simulink model "MySusp_ParasiticFriction_RTW"  (Simulink 9.1)
settings: Solver=ode1  StartTime=0.0  StopTime=inf  FixedStep=0.001  RelTol=1e-3
PreLoadFcn:
  | vehicle = 'Car'; if ~length(which('cmself')), cmenv; end
  | MySusp_ParasiticFriction_RTW_bus
  | MySusp_ParasiticFriction_RTW_params
InitFcn:
  | vehicle = 'Car'; if ~length(which('cmself')), cmenv; end
  | MySusp_ParasiticFriction_RTW_bus
values from neighbouring files (symbols this model uses):
  Damping = 150    [MySusp_ParasiticFriction_RTW_params.m]
  mu_c = 1.0    (= 1)    [MySusp_ParasiticFriction_RTW_params.m]
  PreloadForce = 30    [MySusp_ParasiticFriction_RTW_params.m]
  Stiffness = 50000    [MySusp_ParasiticFriction_RTW_params.m]    (also in MySusp_Spring_RTW_params.m = 5000; MySusp_Stabi_RTW_params.m = 15000)
  v0 = 0.01    [MySusp_ParasiticFriction_RTW_params.m]
Description:
  | CarMaker Plug-in Model Target
settings Model: SuppressorTable=22 serialization::archive 11 0 6 0 0 0 1 0  Creator=ml  LastModifiedBy=ml
settings DataIOCC: SaveFormat=Dataset
settings OptimizationCC: LifeSpan=auto
settings DebuggingCC: UnderspecifiedInitializationDetection=Simplified  MergeDetectMultiDrivingBlocksExec=error  SFUnexpectedBacktrackingDiag=error  SFNoUnconditionalDefaultTransitionDiag=error  SFExecutionAtInitializationDiag=warning
settings HardwareCC: ProdBitPerPointer=64  ProdBitPerSizeT=64  ProdBitPerPtrDiffT=64  ProdLargestAtomicFloat=Float  ProdIntDivRoundTo=Zero  ProdEndianess=LittleEndian  ProdWordSize=64  ProdHWDeviceType=Intel->x86-64 (Windows64)
settings ModelReferenceCC: PropagateSignalLabelsOutOfModel=on
settings RTWCC: SystemTargetFile=CarMaker.tlc  TemplateMakefile=CarMaker_unix-win64.tmf  Description=CarMaker Plug-in Model Target
settings CodeAppCC: MaxIdLength=127
settings STFCustomTargetCC: TargetLangStandard=C99 (ISO)  CombineOutputUpdateFcns=on  MultiInstanceERTCode=on  CodeInterfacePackaging=Reusable function  GRTInterface=off  GenerateAllocFcn=on  SystemTargetFile=CarMaker.tlc
settings GRTTargetCC: TargetLangStandard=C99 (ISO)  ParMdlRefBuildCompliant=off  CompOptLevelCompliant=off  ConcurrentExecutionCompliant=off  CombineOutputUpdateFcns=on  MatFileLogging=off  MultiInstanceERTCode=on  CodeInterfacePackaging=Reusable function  CPPClassGenCompliant=off  GRTInterface=off  GenerateAllocFcn=on  UseToolchainInfoCompliant=off  RTWCAPISignals=on  RTWCAPIParams=on  RTWCAPIStates=on
settings CustomProperty: DataType=string
settings EnumStrPairs: String=Car
settings ConfigComp: CovMetricSettings=dwe  CovHtmlReporting=off  CovSaveCumulativeToWorkspaceVar=off  CovSaveSingleToWorkspaceVar=off  CovExternalEMLEnable=on

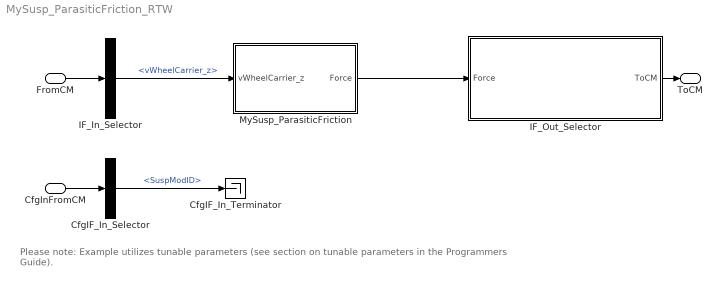
== system MySusp_ParasiticFriction_RTW ==
  note: Please note: Example utilizes tunable parameters (see section on tunable parameters in the Programmers Guide).
  FromCM : Inport  OutDataTypeStr=Bus: cmSusp_ParasiticEffectsIn
  CfgInFromCM : Inport  Port=2  OutDataTypeStr=Bus: cmSusp_ParasiticEffectsCfgIn
  CfgIF_In_Selector : BusSelector  OutputSignals=SuspModID
  CfgIF_In_Terminator : Terminator
  IF_In_Selector : BusSelector  OutputSignals=vWheelCarrier_z
  IF_Out_Selector : Subsystem  mask(Signal Selection){}
      mask help: Signal Selection Block
      settings: OpenFcn=cmSignalSelect('SignalSelection_CB',gcb)
  MySusp_ParasiticFriction : Subsystem
  ToCM : Outport  OutDataTypeStr=Bus: cmSusp_ParasiticEffectsOut
  wires:
  FromCM/1 -> IF_In_Selector/1
  IF_In_Selector/1 -> MySusp_ParasiticFriction/1(vWheelCarrier_z)  "<vWheelCarrier_z>"
  IF_Out_Selector/1(ToCM) -> ToCM/1
  CfgInFromCM/1 -> CfgIF_In_Selector/1
  CfgIF_In_Selector/1 -> CfgIF_In_Terminator/1  "<SuspModID>"
  MySusp_ParasiticFriction/1(Force) -> IF_Out_Selector/1(Force)

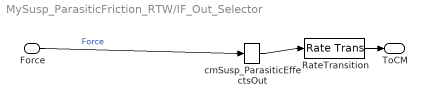
== system MySusp_ParasiticFriction_RTW/IF_Out_Selector ==
  Force : Inport
  RateTransition : RateTransition  OutPortSampleTime=str2num(get_param(bdroot,'FixedStep'))
  cmSusp_ParasiticEffectsOut : BusCreator  Inputs=1
  ToCM : Outport
  wires:
  RateTransition/1 -> ToCM/1
  cmSusp_ParasiticEffectsOut/1 -> RateTransition/1
  Force/1 -> cmSusp_ParasiticEffectsOut/1  "Force"

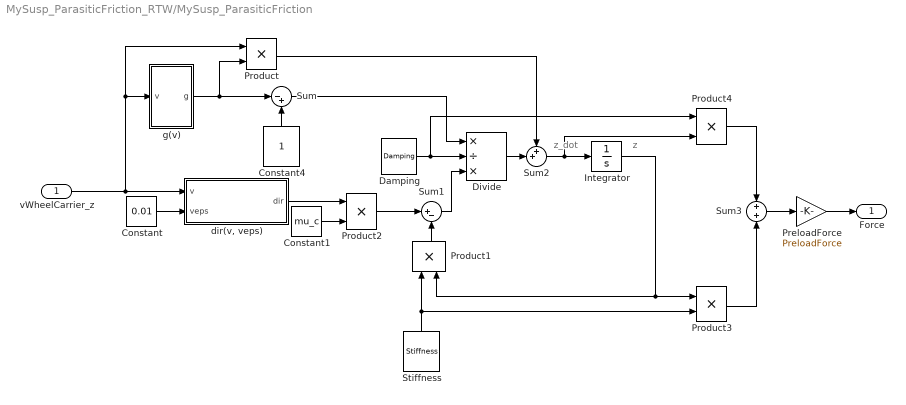
== system MySusp_ParasiticFriction_RTW/MySusp_ParasiticFriction ==
  note: z_dot
  note: z
  vWheelCarrier_z : Inport
  Constant : Constant  Value=0.01
  Constant1 : Constant  Value=mu_c
  Constant4 : Constant
  Damping : Constant  Value=Damping
  Divide : Product  Inputs=*/*
  Integrator : Integrator
  PreloadForce : Gain  Gain=PreloadForce
  Product{,1..4} (5 alike) : Product
  Stiffness : Constant  Value=Stiffness
  Sum : Sum  Inputs=|-+
  Sum1 : Sum  Inputs=|+-
  Sum2 : Sum  Inputs=++|
  Sum3 : Sum
  "dir(v, veps)" : Subsystem
  g(v) : Subsystem
  Force : Outport
  wires:
  Sum3/1 -> PreloadForce/1
  PreloadForce/1 -> Force/1
  Sum/1 -> Divide/1
  Stiffness/1 -> Product1/1, Product3/2
  Sum1/1 -> Divide/3
  Damping/1 -> Product4/1, Divide/2
  Divide/1 -> Sum2/2
  Product/1 -> Sum2/1
  vWheelCarrier_z/1 -> "dir(v, veps)"/1(v), g(v)/1(v), Product/1
  Constant/1 -> "dir(v, veps)"/2(veps)
  g(v)/1(g) -> Sum/1, Product/2
  Constant1/1 -> Product2/2
  "dir(v, veps)"/1(dir) -> Product2/1
  Product2/1 -> Sum1/1
  Constant4/1 -> Sum/2
  Sum2/1 -> Product4/2, Integrator/1
  Integrator/1 -> Product1/2, Product3/1
  Product1/1 -> Sum1/2
  Product3/1 -> Sum3/2
  Product4/1 -> Sum3/1

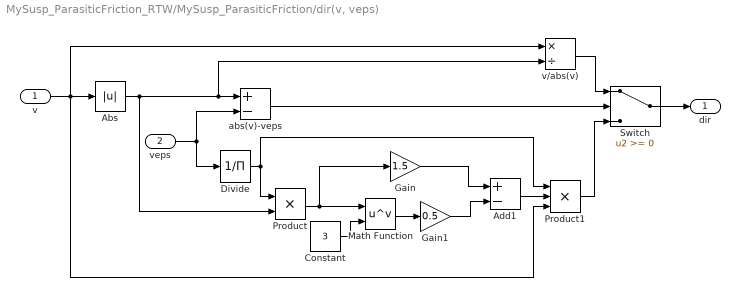
== system MySusp_ParasiticFriction_RTW/MySusp_ParasiticFriction/dir(v, veps) ==
  v : Inport
  veps : Inport  Port=2
  Abs : Abs
  Add1 : Sum  Inputs=+-
  Constant : Constant  Value=3
  Divide : Product  Inputs=/
  Gain : Gain  Gain=1.5
  Gain1 : Gain  Gain=0.5
  Math Function : Math  Operator=pow  SaturateOnIntegerOverflow=on
  Product : Product
  Product1 : Product  Inputs=3
  Switch : Switch
  abs(v)-veps : Sum  Inputs=+-
  v/abs(v) : Product  Inputs=*/
  dir : Outport
  wires:
  v/1 -> v/abs(v)/1, Product1/3, Abs/1
  veps/1 -> Divide/1, abs(v)-veps/2
  Abs/1 -> Product/2, v/abs(v)/2, abs(v)-veps/1
  abs(v)-veps/1 -> Switch/2
  v/abs(v)/1 -> Switch/1
  Switch/1 -> dir/1
  Product/1 -> Gain/1, Math Function/1
  Constant/1 -> Math Function/2
  Math Function/1 -> Gain1/1
  Gain1/1 -> Add1/2
  Gain/1 -> Add1/1
  Add1/1 -> Product1/2
  Product1/1 -> Switch/3
  Divide/1 -> Product1/1, Product/1

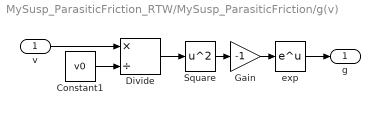
== system MySusp_ParasiticFriction_RTW/MySusp_ParasiticFriction/g(v) ==
  v : Inport
  Constant1 : Constant  Value=v0
  Divide : Product  Inputs=*/
  Gain : Gain  Gain=-1
  Square : Math  Operator=square  SaturateOnIntegerOverflow=on
  exp : Math  SaturateOnIntegerOverflow=on
  g : Outport
  wires:
  v/1 -> Divide/1
  Divide/1 -> Square/1
  exp/1 -> g/1
  Constant1/1 -> Divide/2
  Gain/1 -> exp/1
  Square/1 -> Gain/1
